simulink model "p6"  (R2020a)
settings: Solver=VariableStepAuto  StartTime=0.0  StopTime=10.0  RelTol=1e-3
model workspace (MAT data in the model file):
  g1 = Simulink.Parameter
  g1.Value = 1
  g1.DataType = 'auto'
  g1.Dimensions = [1 1]
  g2 = Simulink.Parameter
  g2.Value = 2
  g2.DataType = 'auto'
  g2.Dimensions = [1 1]
  g3 = Simulink.Parameter
  g3.Value = -3
  g3.DataType = 'auto'
  g3.Dimensions = [1 1]
  g4 = Simulink.Parameter
  g4.Value = -4
  g4.DataType = 'auto'
  g4.Dimensions = [1 1]
  g5 = Simulink.Parameter
  g5.Value = 5
  g5.DataType = 'auto'
  g5.Dimensions = [1 1]
settings Model: Creator=akhil singh  LastModifiedBy=akhil singh

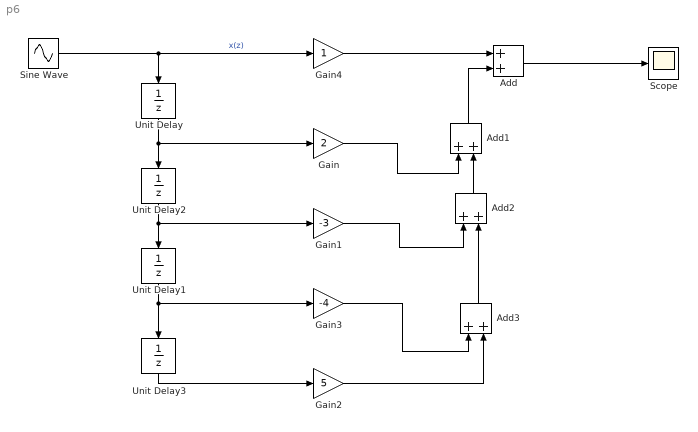
== system p6 ==
  Add{,1..3} (4 alike) : Sum
  Gain : Gain  Gain=2
  Gain1 : Gain  Gain=-3
  Gain2 : Gain  Gain=5
  Gain3 : Gain  Gain=-4
  Gain4 : Gain
  Scope : Scope
  Sine Wave : Sin  SampleTime=0
  Unit Delay{,1..3} (4 alike) : UnitDelay  SampleTime=-1  HasFrameUpgradeWarning=on
  wires:
  Sine Wave/1 -> Unit Delay/1, Gain4/1  "x(z)"
  Gain4/1 -> Add/1
  Unit Delay/1 -> Gain/1, Unit Delay2/1
  Unit Delay2/1 -> Gain1/1, Unit Delay1/1
  Unit Delay1/1 -> Gain3/1, Unit Delay3/1
  Unit Delay3/1 -> Gain2/1
  Gain3/1 -> Add3/1
  Gain2/1 -> Add3/2
  Add3/1 -> Add2/2
  Gain1/1 -> Add2/1
  Add2/1 -> Add1/2
  Gain/1 -> Add1/1
  Add1/1 -> Add/2
  Add/1 -> Scope/1
